simulink subsystem "LQG_Integral"  (R2025b)
settings: Solver=VariableStepAuto  StartTime=0.0  StopTime=10.0  RelTol=1e-3
values from neighbouring files (symbols this model uses):
  K_lqr = lqr(sysdt_bar, Q, R)    [LQG_Integral.m]    (also in LQR_gains_FIR.m = lqr(sysdt_bar, Q_bar, R_bar); LQR_gains_OPT.m = lqr(sysdt_bar, Q_bar, R_bar))
  x0_bar = [E0; P0; T0; zeros(nx+nz-3, 1)]    [LQG_Integral.m]
undefined symbols (not defined in the file or in its folder): DAC_lim_u, DiscIntNeverNeededParam, Discrete, R_kalman, Time, U_e_real
libraries: ctrlSharedLib x1
settings Model: Creator=leeta  LastModifiedBy=leeta

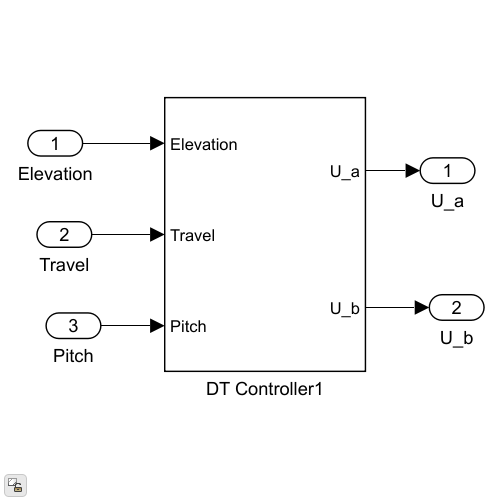
[thumbnail: Simulink's stored preview of the top-level diagram]
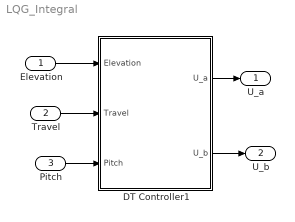
== system LQG_Integral ==
  Elevation : Inport
  Travel : Inport  Port=2
  Pitch : Inport  Port=3
  DT Controller1 : Subsystem
  U_a : Outport
  U_b : Outport  Port=2
  wires:
  Travel/1 -> DT Controller1/2(Travel)
  Elevation/1 -> DT Controller1/1(Elevation)
  DT Controller1/2(U_b) -> U_b/1
  Pitch/1 -> DT Controller1/3(Pitch)
  DT Controller1/1(U_a) -> U_a/1

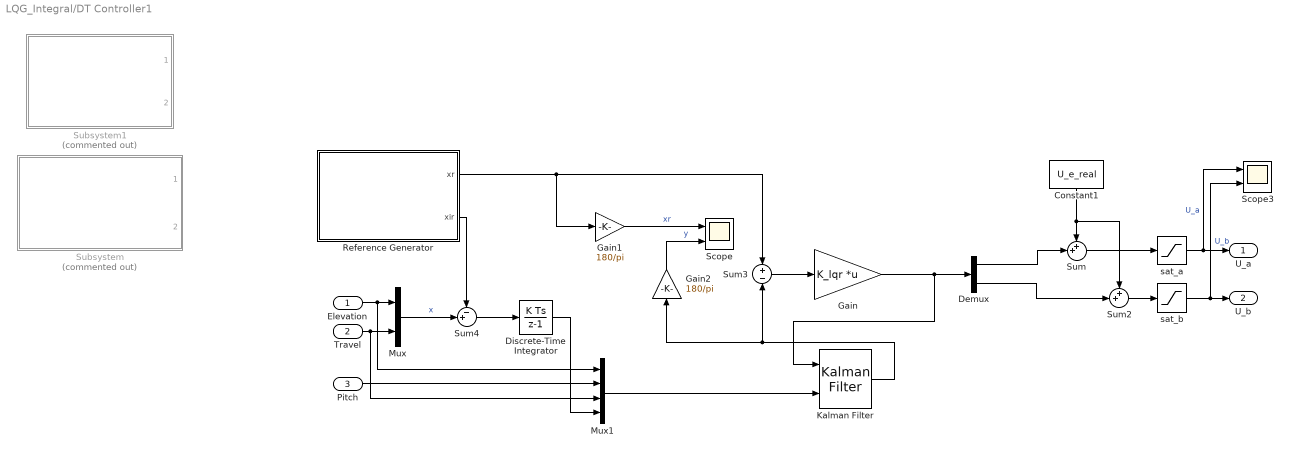
== system LQG_Integral/DT Controller1 ==
  Elevation : Inport
  Travel : Inport  Port=2
  Pitch : Inport  Port=3
  Constant1 : Constant  Value=U_e_real
  Demux : Demux  Outputs=2
  Discrete-Time Integrator : DiscreteIntegrator  SampleTime=-1  ICPrevOutput=DiscIntNeverNeededParam  ICPrevScaledInput=DiscIntNeverNeededParam
  Gain : Gain  Gain=K_lqr  Multiplication=Matrix(K*u)
  Gain1 : Gain  Gain=180/pi
  Gain2 : Gain  Gain=180/pi
  Kalman Filter : ctrlSharedLib/Kalman Filter  TimeDomain=Discrete-Time  UseCurrentEstimator=on  ModelSource=LTI State-Space Variable  ModelSourceVariable=sysdt_bar  A=0.95  B=1  C=1  D=0  NumberOfStates=1  NumberOfInputs=1  NumberOfOutputs=1  InitialEstimateSource=Dialog  X0=x0_bar  P0=10  UseK=off  UseGH=off  NumberOfProcessNoiseInputs=1  G=1  TimeInvariantG=on  H=0  TimeInvariantH=on  Q=1  TimeInvariantQ=on  R=R_kalman  TimeInvariantR=on  N=0  TimeInvariantN=on  AddInputPort=on  AddEnablePort=off  OutputEstimatedY=off  OutputP=off  Ts=-1
  Mux : Mux  Inputs=2
  Mux1 : Mux
  Reference Generator : Subsystem  Variant=on
  Scope : Scope  NumInputPorts=2
      settings: ActiveDisplayYMinimum=-438.65345938128905  ActiveDisplayYMaximum=326.52206894597282
  Scope3 : Scope  NumInputPorts=2
      settings: ActiveDisplayYMinimum=-2.9768524114607064  ActiveDisplayYMaximum=15.395343151144219  DataLoggingVariableName=ScopeData6
  Subsystem : Subsystem  Commented=on  ReferencedSubsystem=FIRReferenceGenerator
  Subsystem1 : Subsystem  Commented=on  ReferencedSubsystem=OptimalReferenceGenerator
  Sum : Sum  Inputs=++|
  Sum2 : Sum  Inputs=++|
  Sum3 : Sum  Inputs=+|-
  Sum4 : Sum  Inputs=-+|
  sat_a : Saturate  UpperLimit=DAC_lim_u  LowerLimit=0
  sat_b : Saturate  UpperLimit=DAC_lim_u  LowerLimit=0
  U_a : Outport
  U_b : Outport  Port=2
  wires:
  Reference Generator/2(xir) -> Sum4/1
  Reference Generator/1(xr) -> Gain1/1, Sum3/1
  Gain2/1 -> Scope/2  "y"
  Gain1/1 -> Scope/1  "xr"
  Discrete-Time Integrator/1 -> Mux1/4
  Sum4/1 -> Discrete-Time Integrator/1
  Mux1/1 -> Kalman Filter/2
  Pitch/1 -> Mux1/2
  Mux/1 -> Sum4/2  "x"
  Sum3/1 -> Gain/1
  Constant1/1 -> Sum/1, Sum2/1
  Sum2/1 -> sat_b/1
  Sum/1 -> sat_a/1
  Demux/2 -> Sum2/2
  Demux/1 -> Sum/2
  Gain/1 -> Demux/1, Kalman Filter/1
  Kalman Filter/1 -> Sum3/2, Gain2/1
  Travel/1 -> Mux/2, Mux1/3
  Elevation/1 -> Mux/1, Mux1/1
  sat_a/1 -> U_a/1, Scope3/1  "U_a"
  sat_b/1 -> U_b/1, Scope3/2  "U_b"

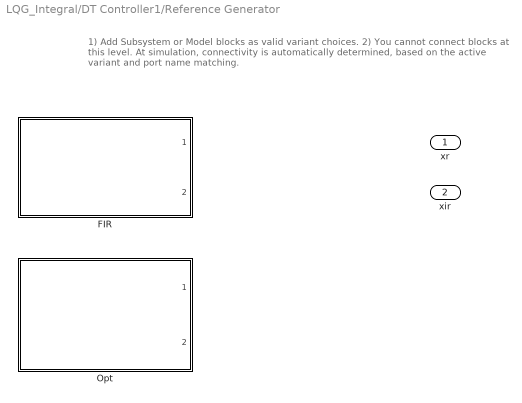
== system LQG_Integral/DT Controller1/Reference Generator ==
  note: 1) Add Subsystem or Model blocks as valid variant choices.
      | 2) You cannot connect blocks at this level. At simulation, connectivity is automatically
      | determined, based on the active variant and port name matching.
  FIR : Subsystem  VariantControl=ref_v ==2  ReferencedSubsystem=FIRReferenceGenerator
  Opt : Subsystem  VariantControl=ref_v==1  ReferencedSubsystem=OptimalReferenceGenerator
  xr : Outport
  xir : Outport  Port=2
